simulink model "mcb_open_loop_control_host_model"  (R2021a)
settings: Solver=FixedStepDiscrete  StartTime=0.0  StopTime=inf  RelTol=1e-3  EnableMultiTasking=on
InitFcn:
  | if( strcmp(get_param([gcs '/TX/HW_Selected'], 'Value'), '0'))
  |       set_param([gcs '/Host Serial Setup'], 'baudRateA', '5.625e6');
  | elseif( strcmp(get_param([gcs '/TX/HW_Selected'], 'Value'), '1'))
  |       set_param([gcs '/Host Serial Setup'], 'baudRateA', '5e6');
  | end
undefined symbols (not defined in the file or in its folder): Ts
libraries: mcbhostblockslib x3
PreSaveFcn:
  | if( strcmp(get_param([gcs '/TX/HW_Selected'], 'Value'), '0'))
  |       set_param([gcs '/Host Serial Setup'], 'baudRateA', '5.625e6');
  | elseif( strcmp(get_param([gcs '/TX/HW_Selected'], 'Value'), '1'))
  |       set_param([gcs '/Host Serial Setup'], 'baudRateA', '5e6');
  | end
settings Model: Creator=The MathWorks, Inc.  LastModifiedBy=The MathWorks, Inc.
settings SolverCC: AlgebraicLoopSolver=TrustRegion
settings DataIOCC: LimitDataPoints=on  SaveFormat=Array  ReturnWorkspaceOutputs=off
settings OptimizationCC: LifeSpan=1  EfficientTunableParamExpr=on
settings DebuggingCC: UnderspecifiedInitializationDetection=Classic  MergeDetectMultiDrivingBlocksExec=none  SolverPrmCheckMsg=warning  ParameterPrecisionLossMsg=none  AllowSymbolicDim=off  PregeneratedLibrarySubsystemCodeDiagnostic=none  SFUnexpectedBacktrackingDiag=warning  SFNoUnconditionalDefaultTransitionDiag=warning  SFExecutionAtInitializationDiag=none  SFMachineParentedDataDiag=warning  ArithmeticOperatorsInVariantConditions=warning
settings HardwareCC: ProdBitPerPointer=32  ProdLargestAtomicFloat=None  ProdIntDivRoundTo=Undefined  ProdEndianess=Unspecified  ProdWordSize=32  ProdHWDeviceType=32-bit Generic
settings ModelReferenceCC: PropagateSignalLabelsOutOfModel=off
settings SFSimCC: SimUseLocalCustomCode=off  MATLABDynamicMemAlloc=off
settings RTWCC: Description=Real-Time Workshop Embedded Coder  SystemTargetFile=ert.tlc  TemplateMakefile=ert_default_tmf  GenerateReport=on  RTWUseLocalCustomCode=off  IncludeHyperlinkInReport=on  LaunchReport=on  GenerateTraceInfo=on  GenerateTraceReport=on  GenerateTraceReportSl=on  GenerateTraceReportSf=on  GenerateTraceReportEml=on
settings CodeAppCC: IgnoreCustomStorageClasses=off  StateflowObjectComments=on  InternalIdentifier=Classic
settings ERTTargetCC: MultiwordLength=2048  GenerateSampleERTMain=on  ERTCustomFileTemplate=example_file_process.tlc  ConvertIfToSwitch=off  SuppressUnreachableDefaultCases=off
settings ConfigComp: CovMetricSettings=dw  CovSaveCumulativeToWorkspaceVar=on  CovSaveSingleToWorkspaceVar=on  CovExternalEMLEnable=off  CovSFcnEnable=off

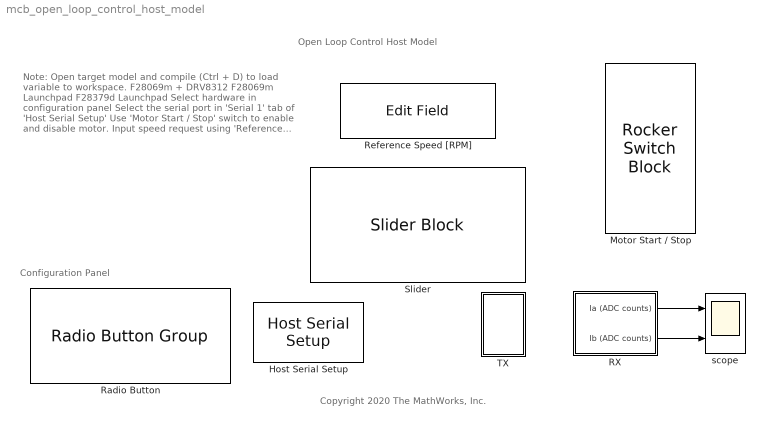
== system mcb_open_loop_control_host_model ==
  note: Note:
      | Open target model and compile (Ctrl + D) to load variable to workspace.
      | F28069m + DRV8312
      | F28069m Launchpad
      | F28379d Launchpad
      | Select hardware in configuration panel
      | Select the serial port in 'Serial 1' tab of 'Host Serial Setup'
      | Use 'Motor Start / Stop' switch to enable and disable motor.
      | Input speed request using 'Reference Speed' text box or sliding bar.
      | Observe the ADC counts for phase current measurent in scope
  note: Open Loop Control Host Model
  note: Copyright 2020 The MathWorks, Inc.
  note: Configuration Panel
  Host Serial Setup : mcbhostblockslib/Host Serial Setup  Priority=-99  comPortSer1='Please_select_a_port'  baudRateA=5.625e6  charLenA=8  stopBitA=1  parityA=none  timeoutA=2  ByteOrderA=LittleEndian  comPortSer2='Please_select_a_port'  baudRateB=115200  charLenB=8  stopBitB=1  parityB=none  timeoutB=1.0  ByteOrderB=LittleEndian  comPortSer3='Please_select_a_port'  baudRateC=115200  charLenC=8  stopBitC=1  parityC=none  timeoutC=1.0  ByteOrderC=LittleEndian  comPortSer4='Please_select_a_port'  baudRateD=115200  charLenD=8  stopBitD=1  parityD=none  timeoutD=1.0  ByteOrderD=LittleEndian
      settings: SourceProductBaseCode=MT
  Motor Start / Stop : RockerSwitchBlock  LabelPosition=Hide
      settings: Values={{'On', 'Off'}, [1 0]}
  RX : Subsystem
  Radio Button : RadioButtonGroup  LabelPosition=Hide  SelectedLabel=TI F28069M  ButtonGroupName=Group
      settings: Values={{'TI F28069M', 'TI F28379D'}, [0 1]}
  Reference Speed [RPM] : EditField  LabelPosition=Hide  ShowInitialText=on  Alignment=Center
  Slider : SliderBlock  LabelPosition=Hide  ScaleMin=-2000  ScaleMax=2000
  TX : Subsystem
  scope : Scope  NumInputPorts=2
  wires:
  RX/1(Ia (ADC counts)) -> scope/1
  RX/2(Ib (ADC counts)) -> scope/2

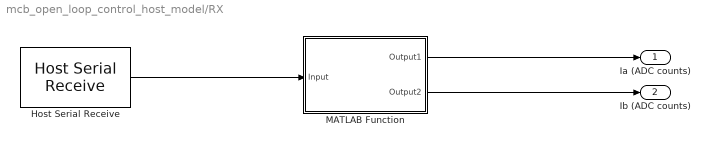
== system mcb_open_loop_control_host_model/RX ==
  Host Serial Receive : mcbhostblockslib/Host Serial Receive  serialCon=Serial 1  dataHead='SS'  dataTail='EE'  dataType=uint16  dataDim=[600 2]  initValue=0  errOption=Output the last received value  errValue=0  sampleTime=600 * Ts  outputStatus=off  blockingMode=on
      settings: SourceProductBaseCode=MT
  MATLAB Function : MATLAB Function  TreatAsAtomicUnit=on
  Ia (ADC counts) : Outport
  Ib (ADC counts) : Outport  Port=2
  wires:
  MATLAB Function/2(Output2) -> Ib (ADC counts)/1
  MATLAB Function/1(Output1) -> Ia (ADC counts)/1
  Host Serial Receive/1 -> MATLAB Function/1(Input)

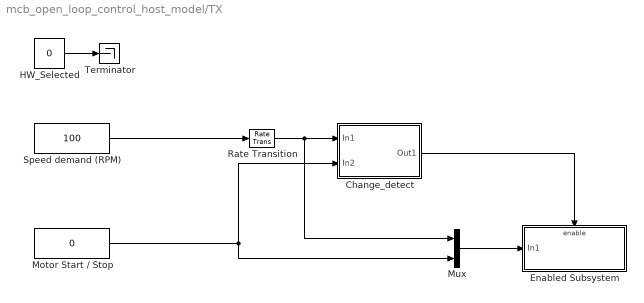
== system mcb_open_loop_control_host_model/TX ==
  Change_detect : Subsystem
  Enabled Subsystem : Subsystem  TreatAsAtomicUnit=on
  HW_Selected : Constant  Value=0  OutDataTypeStr=uint8
  Motor Start / Stop : Constant  Value=0  VectorParams1D=off  OutDataTypeStr=single  SampleTime=0.03
  Mux : Mux  Inputs=2
  Rate Transition : RateTransition  OutPortSampleTime=0.03
  Speed demand (RPM) : Constant  Value=100  VectorParams1D=off  OutDataTypeStr=single  SampleTime=0.03
  Terminator : Terminator
  wires:
  Motor Start / Stop/1 -> Mux/2, Change_detect/2(In2)
  Speed demand (RPM)/1 -> Rate Transition/1
  Mux/1 -> Enabled Subsystem/1(In1)
  Rate Transition/1 -> Mux/1, Change_detect/1(In1)
  Change_detect/1(Out1) -> Enabled Subsystem/Enable
  HW_Selected/1 -> Terminator/1

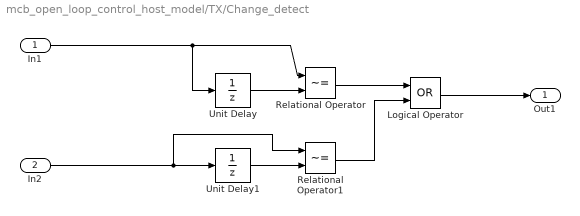
== system mcb_open_loop_control_host_model/TX/Change_detect ==
  In1 : Inport
  In2 : Inport  Port=2
  Logical Operator : Logic  Operator=OR  AllPortsSameDT=off  OutDataTypeStr=boolean
  Relational Operator : RelationalOperator  Operator=~=  OutDataTypeStr=boolean  RndMeth=Nearest
  Relational Operator1 : RelationalOperator  Operator=~=  OutDataTypeStr=boolean  RndMeth=Nearest
  Unit Delay : UnitDelay  InitialCondition=0.5  SampleTime=-1  HasFrameUpgradeWarning=on
  Unit Delay1 : UnitDelay  SampleTime=-1  HasFrameUpgradeWarning=on
  Out1 : Outport  VectorParamsAs1DForOutWhenUnconnected=off
  wires:
  In2/1 -> Relational Operator1/1, Unit Delay1/1
  Relational Operator1/1 -> Logical Operator/2
  Unit Delay1/1 -> Relational Operator1/2
  Unit Delay/1 -> Relational Operator/2
  In1/1 -> Unit Delay/1, Relational Operator/1
  Relational Operator/1 -> Logical Operator/1
  Logical Operator/1 -> Out1/1

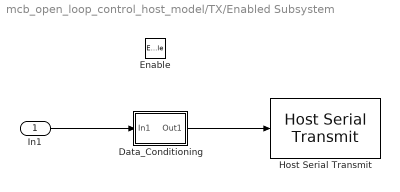
== system mcb_open_loop_control_host_model/TX/Enabled Subsystem ==
  In1 : Inport
  Enable : EnablePort
  Data_Conditioning : Subsystem
  Host Serial Transmit : mcbhostblockslib/Host Serial Transmit  serialCon=Serial 1  header=''  tail=''  enableBlockingMode=off
      settings: SourceProductBaseCode=MT
  wires:
  In1/1 -> Data_Conditioning/1(In1)
  Data_Conditioning/1(Out1) -> Host Serial Transmit/1

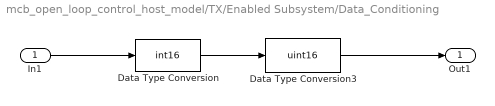
== system mcb_open_loop_control_host_model/TX/Enabled Subsystem/Data_Conditioning ==
  In1 : Inport
  Data Type Conversion : DataTypeConversion  OutDataTypeStr=int16  RndMeth=Simplest
  Data Type Conversion3 : DataTypeConversion  OutDataTypeStr=uint16  ConvertRealWorld=Stored Integer (SI)  RndMeth=Simplest
  Out1 : Outport  VectorParamsAs1DForOutWhenUnconnected=off
  wires:
  In1/1 -> Data Type Conversion/1
  Data Type Conversion3/1 -> Out1/1
  Data Type Conversion/1 -> Data Type Conversion3/1

== matlab function mcb_open_loop_control_host_model/RX/MATLAB Function ==
  data: Output1 output; Output2 output; Input input
function [ Output1, Output2] = unBuf(Input)

Output1= Input(:, 1);
Output2 = Input(:, 2);
end
